simulink model "square_or_not_square"  (R2021b)
settings: Solver=FixedStepAuto  StartTime=0.0  StopTime=10.0  FixedStep=0.01  RelTol=1e-3
settings Model: Creator=Xavier  LastModifiedBy=Xavier

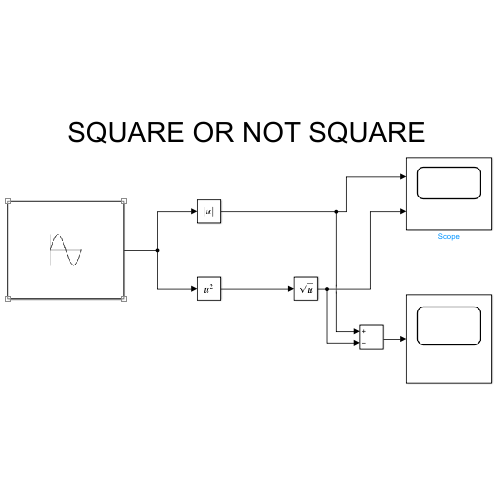
[thumbnail: Simulink's stored preview of the top-level diagram]
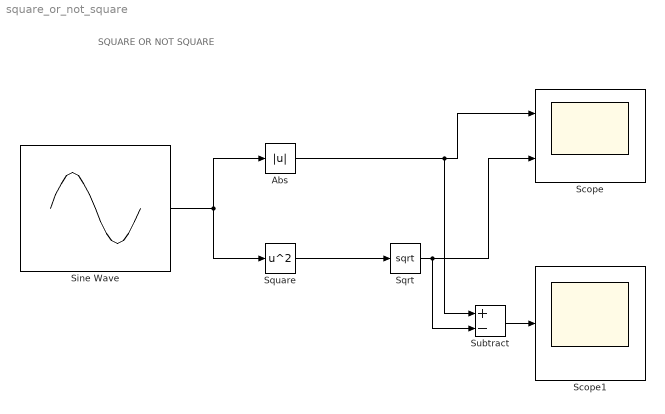
== system square_or_not_square ==
  note: SQUARE OR NOT SQUARE
  Abs : Abs
  Scope : Scope  NumInputPorts=2
  Scope1 : Scope
  Sine Wave : Sin  SampleTime=0
  Sqrt : Sqrt  SaturateOnIntegerOverflow=on
  Square : Math  Operator=square  SaturateOnIntegerOverflow=on
  Subtract : Sum  Inputs=+-
  wires:
  Sine Wave/1 -> Square/1, Abs/1
  Square/1 -> Sqrt/1
  Abs/1 -> Subtract/1, Scope/1
  Sqrt/1 -> Subtract/2, Scope/2
  Subtract/1 -> Scope1/1
